simulink model "Sim1"  (R2022a)
settings: Solver=VariableStepAuto  StartTime=0.0  StopTime=10.0  RelTol=1e-3
libraries: dspadpt3 x1
settings Model: Creator=targi  LastModifiedBy=targi

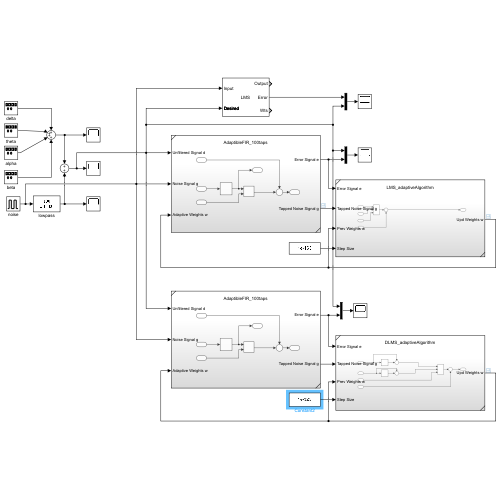
[thumbnail: Simulink's stored preview of the top-level diagram]
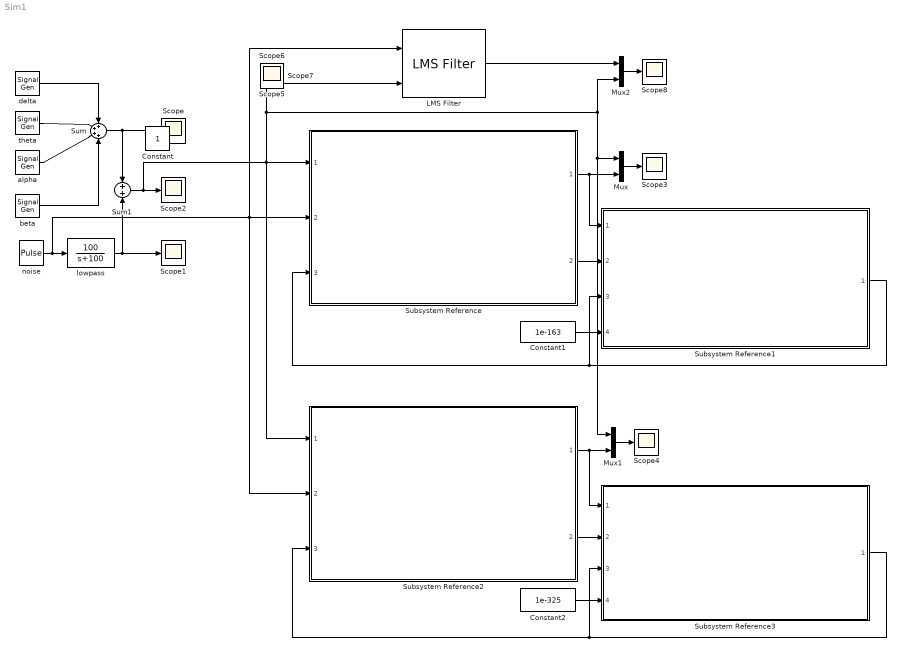
== system Sim1 ==
  Constant1 : Constant  Value=1e-163
  Constant2 : Constant  Value=1e-325
  LMS Filter : dspadpt3/LMS Filter  Algo=LMS  L=50  stepflag=Dialog  mu=1e-1  leakage=1.0  ic=0  Adapt=off  resetflag=None  weights=on  addnparflag=off  roundingMode=Floor  overflowMode=off
      settings: SourceProductBaseCode=DS
  Mux : Mux  Inputs=2
  Mux1 : Mux  Inputs=2
  Mux2 : Mux  Inputs=2
  Scope{,1..8} (9 alike) : Scope
  Subsystem Reference : Subsystem  ReferencedSubsystem=AdaptibleFIR_100taps
  Subsystem Reference1 : Subsystem  ReferencedSubsystem=LMS_adaptiveAlgorithm
  Subsystem Reference2 : Subsystem  ReferencedSubsystem=AdaptibleFIR_100taps
  Subsystem Reference3 : Subsystem  ReferencedSubsystem=DLMS_adaptiveAlgorithm
  Sum : Sum  Inputs=++++
  Sum1 : Sum  Inputs=+|+
  alpha : SignalGenerator  Amplitude=.002  Frequency=10
  beta : SignalGenerator  Amplitude=.001  Frequency=22
  delta : SignalGenerator  Amplitude=.004  Frequency=2
  lowpass : TransferFcn  Numerator=[100]  Denominator=[1 100]
  noise : DiscretePulseGenerator  PulseType=Time based  Period=.4  PulseWidth=5
  theta : SignalGenerator  Amplitude=.003  Frequency=6
  Constant : Constant  IOType=siggen
  wires:
  Subsystem Reference/2 -> Subsystem Reference1/2
  Subsystem Reference/1 -> Subsystem Reference1/1, Mux/2
  Subsystem Reference1/1 -> Subsystem Reference/3, Subsystem Reference1/3
  Subsystem Reference2/2 -> Subsystem Reference3/2
  Subsystem Reference2/1 -> Mux1/2, Subsystem Reference3/1
  Subsystem Reference3/1 -> Subsystem Reference2/3, Subsystem Reference3/3
  Constant1/1 -> Subsystem Reference1/4
  Constant2/1 -> Subsystem Reference3/4
  delta/1 -> Sum/1
  theta/1 -> Sum/2
  alpha/1 -> Sum/3
  beta/1 -> Sum/4
  Sum/1 -> Scope/1, Sum1/1
  noise/1 -> Subsystem Reference2/2, LMS Filter/1, Subsystem Reference/2, lowpass/1
  lowpass/1 -> Scope1/1, Sum1/2
  Sum1/1 -> Subsystem Reference2/1, LMS Filter/2, Mux1/1, Mux/1, Mux2/2, Subsystem Reference/1, Scope2/1
  Mux/1 -> Scope3/1
  Mux1/1 -> Scope4/1
  Mux2/1 -> Scope8/1
  LMS Filter/2 -> Mux2/1
